simulink model "Controller"  (R2019b)
settings: Solver=VariableStepAuto  StartTime=0.0  StopTime=10.0  RelTol=1e-3
values from neighbouring files (symbols this model uses):
  Mech_Vent_pressure = 17    [Mech_vent_test.m]
  NM_block_gain = 1    [Mech_vent_test.m]
  PIO2 = 150    [Dead_Space_Khoo_IC.m]    (also in Gas_Exchange_IC.m; Respiratory_IC.m)
  PIO2_change = -90    [Mech_vent_test.m]    (also in Respiratory_IC.m = 0)
  t_Mech_Vent_duration = 0    [Mech_vent_test.m]
  t_Mech_Vent_start = 0    [Mech_vent_test.m]
  t_NM_block_duration = 0    [Mech_vent_test.m]
  t_NM_block_start = 0    [Mech_vent_test.m]
  t_O2_duration = 0    [Mech_vent_test.m]    (also in Respiratory_IC.m)
  t_O2_start = 0    [Mech_vent_test.m]    (also in Respiratory_IC.m)
  Ventilator_rate = 12    [Mech_vent_test.m]
settings Model: Creator=z9070419  LastModifiedBy=z9070419

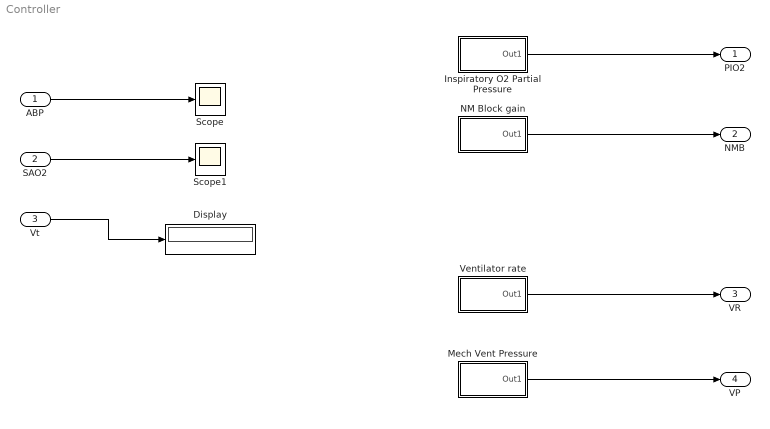
== system Controller ==
  ABP : Inport
  SAO2 : Inport  Port=2
  Vt : Inport  Port=3
  Display : Display
  Inspiratory O2 Partial Pressure : Subsystem  mask{begin_time=t_O2_start, end_time=t_O2_start+t_O2_duration, init_value=PIO2, final_value=PIO2+PIO2_change}
      mask prompts: begin_time "pulse begin"; end_time "pulse end"; init_value "initial value"; final_value "final value"
      mask Display: disp('pulse')
  Mech Vent Pressure : Subsystem  mask{begin_time=t_Mech_Vent_start, end_time=t_Mech_Vent_start+t_Mech_Vent_duration, init_value=0, final_value=Mech_Vent_pressure}
      mask prompts: begin_time "pulse begin"; end_time "pulse end"; init_value "initial value"; final_value "final value"
      mask Display: disp('pulse')
  NM Block gain : Subsystem  mask{begin_time=t_NM_block_start, end_time=t_NM_block_start+t_NM_block_duration, NM_block_gain=NM_block_gain}
      mask prompts: begin_time "pulse begin"; end_time "pulse end"; NM_block_gain "neuromuscular block gain"
      mask Display: disp('pulse')
  Scope : Scope
  Scope1 : Scope
  Ventilator rate : Subsystem  mask{begin_time=t_Mech_Vent_start, end_time=t_Mech_Vent_start+t_Mech_Vent_duration, Ventilator_rate=Ventilator_rate}
      mask prompts: begin_time "pulse begin"; end_time "pulse end"; Ventilator_rate "ventilator rate"
      mask Display: disp('pulse')
  PIO2 : Outport
  NMB : Outport  Port=2
  VR : Outport  Port=3
  VP : Outport  Port=4
  wires:
  Ventilator rate/1(Out1) -> VR/1
  Mech Vent Pressure/1(Out1) -> VP/1
  NM Block gain/1(Out1) -> NMB/1
  Inspiratory O2 Partial Pressure/1(Out1) -> PIO2/1
  ABP/1 -> Scope/1
  SAO2/1 -> Scope1/1
  Vt/1 -> Display/1

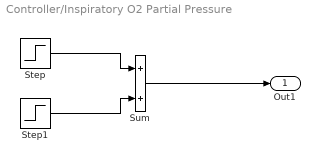
== system Controller/Inspiratory O2 Partial Pressure ==
  Step : Step  Time=begin_time  Before=init_value  After=final_value  SampleTime=0
  Step1 : Step  Time=end_time  After=init_value-final_value  SampleTime=0
  Sum : Sum  Inputs=|++  SaturateOnIntegerOverflow=on  InputSameDT=on  OutDataTypeStr=Inherit: Same as first input
  Out1 : Outport
  wires:
  Sum/1 -> Out1/1
  Step1/1 -> Sum/2
  Step/1 -> Sum/1

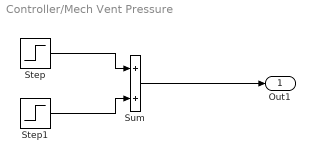
== system Controller/Mech Vent Pressure ==
  Step : Step  Time=begin_time  Before=init_value  After=final_value  SampleTime=0
  Step1 : Step  Time=end_time  After=init_value-final_value  SampleTime=0
  Sum : Sum  Inputs=|++  SaturateOnIntegerOverflow=on  InputSameDT=on  OutDataTypeStr=Inherit: Same as first input
  Out1 : Outport
  wires:
  Step/1 -> Sum/1
  Step1/1 -> Sum/2
  Sum/1 -> Out1/1

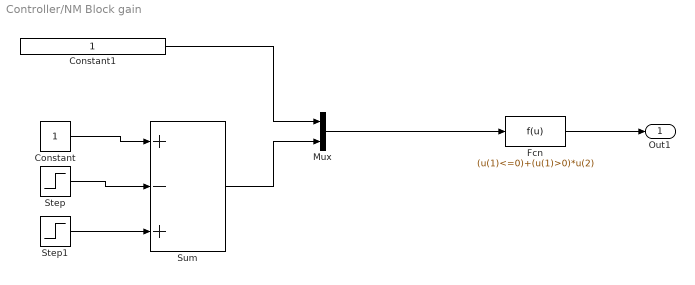
== system Controller/NM Block gain ==
  Constant : Constant
  Constant1 : Constant
  Fcn : Fcn  Expr=(u(1)<=0)+(u(1)>0)*u(2)
  Mux : Mux  Inputs=2
  Step : Step  Time=begin_time  After=NM_block_gain  SampleTime=0
  Step1 : Step  Time=end_time  After=NM_block_gain  SampleTime=0
  Sum : Sum  Inputs=+-+  SaturateOnIntegerOverflow=on  InputSameDT=on  OutDataTypeStr=Inherit: Same as first input
  Out1 : Outport
  wires:
  Step/1 -> Sum/2
  Step1/1 -> Sum/3
  Constant/1 -> Sum/1
  Fcn/1 -> Out1/1
  Sum/1 -> Mux/2
  Constant1/1 -> Mux/1
  Mux/1 -> Fcn/1

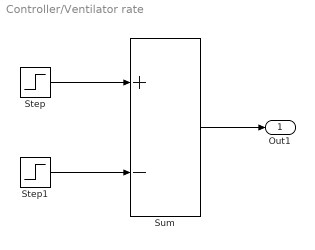
== system Controller/Ventilator rate ==
  Step : Step  Time=begin_time  After=Ventilator_rate  SampleTime=0
  Step1 : Step  Time=end_time  After=Ventilator_rate  SampleTime=0
  Sum : Sum  Inputs=+-  SaturateOnIntegerOverflow=on  InputSameDT=on  OutDataTypeStr=Inherit: Same as first input
  Out1 : Outport
  wires:
  Step/1 -> Sum/1
  Step1/1 -> Sum/2
  Sum/1 -> Out1/1
